simulink model "LoopCounterUpdateTimeModel"  (R2022b)
settings: Solver=VariableStepAuto  StartTime=0.0  StopTime=10.0  RelTol=1e-3
libraries: simulink x2
settings Model: Creator=ferbe  LastModifiedBy=ferbe

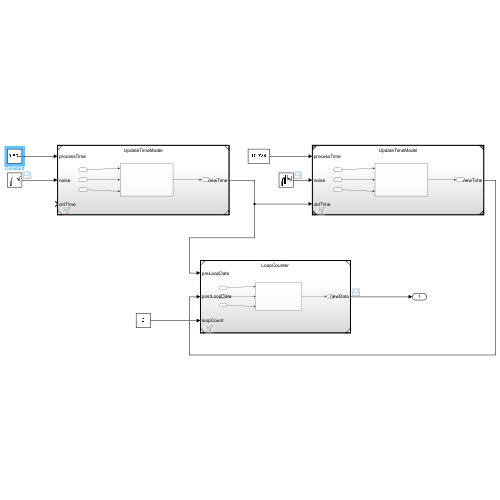
[thumbnail: Simulink's stored preview of the top-level diagram]
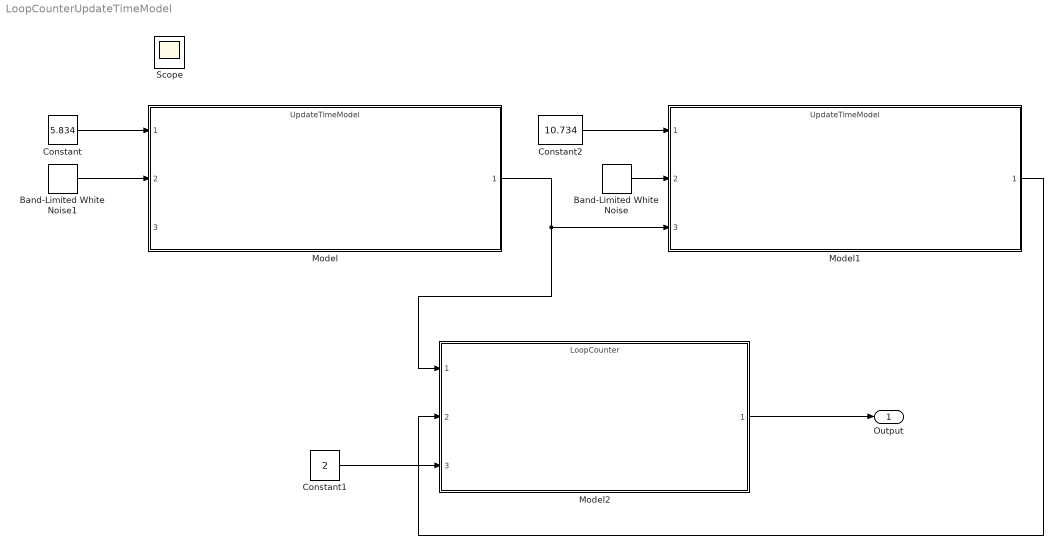
== system LoopCounterUpdateTimeModel ==
  Band-Limited White Noise : simulink/Sources/Band-Limited White Noise  Cov=[0.1]  Ts=0.1  seed=[23341]
  Band-Limited White Noise1 : simulink/Sources/Band-Limited White Noise  Cov=[0.1]  Ts=0.1  seed=[23341]
  Constant : Constant  Value=5.834
  Constant1 : Constant  Value=2
  Constant2 : Constant  Value=10.734
  Model : ModelReference  ModelNameDialog=UpdateTimeModel.slx  SimulationMode=Normal  ModelReferenceVersion=1.1
  Model1 : ModelReference  ModelNameDialog=UpdateTimeModel.slx  SimulationMode=Normal  ModelReferenceVersion=1.1
  Model2 : ModelReference  ModelNameDialog=LoopCounter.slx  SimulationMode=Normal  ModelReferenceVersion=1.1
  Output : Outport
  Scope : Scope
  wires:
  Band-Limited White Noise/1 -> Model1/2
  Band-Limited White Noise1/1 -> Model/2
  Model2/1 -> Output/1
  Constant2/1 -> Model1/1
  Model/1 -> Model2/1, Model1/3
  Model1/1 -> Model2/2
  Constant1/1 -> Model2/3
  Constant/1 -> Model/1
